simulink model "Model_6DOF"  (R2022b)
settings: Solver=VariableStepAuto  StartTime=0.0  StopTime=SimTime  RelTol=1e-6
InitFcn:
  | INIT_DATA
values from neighbouring files (symbols this model uses):
  g = 9.81    [aero_guid_dat.m]
  K_r = -0.02    [aero_guid_dat.m]
undefined symbols (not defined in the file or in its folder): a_L_c_max, a_N_c_max, b, C_bar, C_D_0, C_D_0_bar, C_D_alpha, C_D_d_e, C_L_0, C_L_0_bar, C_L_alpha, C_l_beta, C_l_d_a, C_L_d_e, C_l_d_r, C_l_p, C_L_q, C_l_r, C_m_0, C_m_alpha, C_m_d_e, C_m_q, C_n_beta, C_n_d_a, C_n_d_r, C_n_p, C_n_r, C_y_beta, C_y_d_a, C_y_d_r, C_y_p, C_y_r, d_T, da_max, da_rate_max, de_max, de_rate_max, dr_max, dr_rate_max, E, EA0, eR_0_IhI_Ih, eS_0_BE_Lh, eV_0_BE_Lh, G_cp, G_I, G_M, G_M_I, G_R, G_s, GC, I, INS_bias_f, INS_bias_omega, INS_imbalance_error, INS_scale_factor_error_f, INS_scale_factor_error_omega, k, K_beta, K_p ... (+34)
libraries: dspsrcs4 x11, matrix_library x6, simulink x5, sharedutil x3, aerolibasang x3, sharedtransform x2, simulink_extras x1, slpidlib x1
(part 2 of 2)

== system Model_6DOF/Airframe/Forces and Moments (in Body)/Gravitational Acceleration ==
  T_BL : Inport
  Constant3 : Constant  Value=g
  Gain1 : Gain  Gain=[ 0 0 1]
  Product1 : Product  Multiplication=Matrix(*)
  Reshape : Reshape  OutputDimensionality=Column vector (2-D)
  g : Outport
  wires:
  Constant3/1 -> Gain1/1
  Gain1/1 -> Reshape/1
  Product1/1 -> g/1  "Gravitational Acceleration components in body"
  Reshape/1 -> Product1/2
  T_BL/1 -> Product1/1

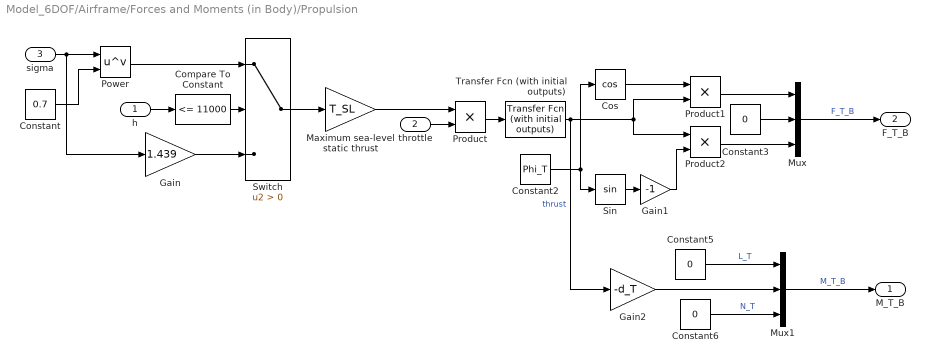
== system Model_6DOF/Airframe/Forces and Moments (in Body)/Propulsion ==
  h : Inport
  throttle : Inport  Port=2
  sigma : Inport  Port=3
  Compare To Constant : simulink/Logic and Bit Operations/Compare To Constant  relop=<=  const=11000  OutDataTypeStr=boolean
  Constant : Constant  Value=0.7
  Constant2 : Constant  Value=Phi_T
  Constant3 : Constant  Value=0
  Constant5 : Constant  Value=0
  Constant6 : Constant  Value=0
  Cos : Trigonometry  Operator=cos
  Gain : Gain  Gain=1.439
  Gain1 : Gain  Gain=-1
  Gain2 : Gain  Gain=-d_T
  Maximum sea-level static thrust : Gain  Gain=T_SL
  Mux : Mux  Inputs=3
  Mux1 : Mux  Inputs=3
  Power : Math  Operator=pow
  Product : Product
  Product1 : Product
  Product2 : Product
  Sin : Trigonometry
  Switch : Switch  Criteria=u2 > Threshold  SaturateOnIntegerOverflow=off  InputSameDT=off
  Transfer Fcn (with initial outputs) : simulink_extras/Additional Linear/Transfer Fcn (with initial outputs)  N=[1]  D=[tau_engine 1]  Y0=TI  U0=0
  M_T_B : Outport
  F_T_B : Outport  Port=2
  wires:
  throttle/1 -> Product/2
  sigma/1 -> Gain/1, Power/1
  Constant/1 -> Power/2
  Maximum sea-level static thrust/1 -> Product/1
  Product/1 -> Transfer Fcn (with initial outputs)/1
  Transfer Fcn (with initial outputs)/1 -> Product1/2, Product2/1, Gain2/1  "thrust"
  Compare To Constant/1 -> Switch/2
  Power/1 -> Switch/1
  h/1 -> Compare To Constant/1
  Switch/1 -> Maximum sea-level static thrust/1
  Gain/1 -> Switch/3
  Constant2/1 -> Sin/1, Cos/1
  Mux/1 -> F_T_B/1  "F_T_B"
  Constant3/1 -> Mux/2
  Product1/1 -> Mux/1
  Product2/1 -> Mux/3
  Cos/1 -> Product1/1
  Sin/1 -> Gain1/1
  Gain1/1 -> Product2/2
  Constant5/1 -> Mux1/1  "L_T"
  Constant6/1 -> Mux1/3  "N_T"
  Mux1/1 -> M_T_B/1  "M_T_B"
  Gain2/1 -> Mux1/2

== system Model_6DOF/Autopilot (Control system)/Acceleration Autopilot/Acceleration Autopilot ==
  a_N_c : Inport
  In Bus Element : Inport  Port=2  PortName=INS_Data  Element=f_sp_B
  In Bus Element1 : Inport  Port=2  PortName=INS_Data  Element=pqr
  Add : Sum  Inputs=+-
  Add1 : Sum  Inputs=--
  Add2 : Sum  Inputs=+-
  Gain : Gain  Gain=-g
  Gain1 : Gain  Gain=G_R
  Gain2 : Gain  Gain=G_I
  Gain3 : Gain  Gain=K_q
  Gain4 : Gain  Gain=-1
  Integrator : Integrator
  Saturation : Saturate  UpperLimit=de_max  LowerLimit=-de_max
  Saturation1 : Saturate  UpperLimit=a_N_c_max  LowerLimit=-a_N_c_max
  Saturation2 : Saturate  UpperLimit=q_c_max  LowerLimit=-q_c_max
  Selector : Selector  InputPortWidth=3  IndexOptions=Index vector (dialog)  Indices=3  OutputSizes=1
  Selector1 : Selector  InputPortWidth=3  IndexOptions=Index vector (dialog)  Indices=2  OutputSizes=1
  d_e_c : Outport
  wires:
  Gain/1 -> Add/1
  Selector/1 -> Add/2
  Add/1 -> Gain2/1, Gain1/1
  Gain2/1 -> Integrator/1
  Gain1/1 -> Add1/1
  Integrator/1 -> Add1/2
  Add2/1 -> Saturation/1
  Saturation/1 -> Gain4/1
  Saturation1/1 -> Gain/1
  Add1/1 -> Saturation2/1  "q_c"
  Saturation2/1 -> Add2/1
  a_N_c/1 -> Saturation1/1
  In Bus Element/1 -> Selector/1
  In Bus Element1/1 -> Selector1/1
  Selector1/1 -> Gain3/1  "q"
  Gain3/1 -> Add2/2
  Gain4/1 -> d_e_c/1

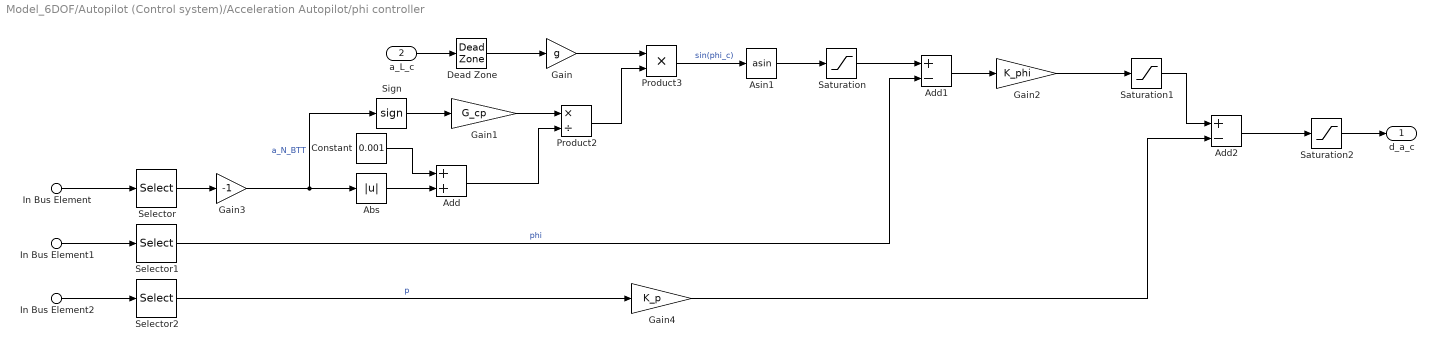
== system Model_6DOF/Autopilot (Control system)/Acceleration Autopilot/phi controller ==
  In Bus Element : Inport  PortName=INS_Data  Element=f_sp_B
  In Bus Element1 : Inport  PortName=INS_Data  Element=phi_theta_psi
  In Bus Element2 : Inport  PortName=INS_Data  Element=pqr
  a_L_c : Inport  Port=2
  Abs : Abs  SaturateOnIntegerOverflow=off
  Add : Sum
  Add1 : Sum  Inputs=+-
  Add2 : Sum  Inputs=+-
  Asin1 : Trigonometry  Operator=asin
  Constant : Constant  Value=0.001
  Dead Zone : DeadZone  LowerValue=-0.01*g  UpperValue=0.01*g
  Gain : Gain  Gain=g
  Gain1 : Gain  Gain=G_cp
  Gain2 : Gain  Gain=K_phi
  Gain3 : Gain  Gain=-1
  Gain4 : Gain  Gain=K_p
  Product2 : Product  Inputs=*/
  Product3 : Product
  Saturation : Saturate  UpperLimit=phi_c_max  LowerLimit=-phi_c_max
  Saturation1 : Saturate  UpperLimit=p_c_max  LowerLimit=-p_c_max
  Saturation2 : Saturate  UpperLimit=da_max  LowerLimit=-da_max
  Selector : Selector  InputPortWidth=3  IndexOptions=Index vector (dialog)  Indices=3  OutputSizes=1
  Selector1 : Selector  InputPortWidth=3  IndexOptions=Index vector (dialog)  Indices=1  OutputSizes=1
  Selector2 : Selector  InputPortWidth=3  IndexOptions=Index vector (dialog)  Indices=1  OutputSizes=1
  Sign : Signum
  d_a_c : Outport
  wires:
  Product3/1 -> Asin1/1  "sin(phi_c)"
  Asin1/1 -> Saturation/1
  Gain3/1 -> Sign/1, Abs/1  "a_N_BTT"
  Gain/1 -> Product3/1
  Sign/1 -> Gain1/1
  Gain1/1 -> Product2/1
  Add/1 -> Product2/2
  Dead Zone/1 -> Gain/1
  Abs/1 -> Add/2
  Product2/1 -> Product3/2
  a_L_c/1 -> Dead Zone/1
  Selector/1 -> Gain3/1
  Constant/1 -> Add/1
  In Bus Element/1 -> Selector/1
  Saturation/1 -> Add1/1
  In Bus Element1/1 -> Selector1/1
  Selector1/1 -> Add1/2  "phi"
  In Bus Element2/1 -> Selector2/1
  Add1/1 -> Gain2/1
  Gain2/1 -> Saturation1/1
  Selector2/1 -> Gain4/1  "p"
  Gain4/1 -> Add2/2
  Add2/1 -> Saturation2/1
  Saturation1/1 -> Add2/1
  Saturation2/1 -> d_a_c/1

== system Model_6DOF/Autopilot (Control system)/Mach Hold Autopilot/throttle required ==
  h : Inport
  alpha : Inport  Port=2
  M_c : Inport  Port=3
  Atmosphere : MATLAB Function  TreatAsAtomicUnit=on
  Constant : Constant  Value=C_D_0_bar
  Constant2 : Constant  Value=C_L_0_bar
  Cos : Trigonometry  Operator=cos
  "Dynamic Pressure " : aerolibasang/Dynamic Pressure
  Gain : Gain  Gain=C_L_alpha
  Gain1 : Gain  Gain=[1;0;0]
  Gain2 : Gain  Gain=k
  Gain3 : Gain  Gain=S
  Product : Product
  Product1 : Product
  Product2 : Product
  Product4 : Product  Inputs=*/
  Scope1 : Scope
  Subtract : Sum
  Subtract1 : Sum
  thrust2trrottle : Subsystem
  throttle_req : Outport
  wires:
  h/1 -> Atmosphere/1(h), thrust2trrottle/1(h)
  M_c/1 -> Product/1
  Atmosphere/2(a) -> Product/2
  Subtract1/1 -> Product1/1, Product1/2  "C_L"
  Constant2/1 -> Subtract1/2
  Constant/1 -> Subtract/1
  Gain2/1 -> Subtract/2
  Subtract/1 -> Product2/2  "C_D"
  Gain/1 -> Subtract1/1
  Product1/1 -> Gain2/1
  alpha/1 -> Cos/1, Gain/1
  Atmosphere/1(rho) -> "Dynamic Pressure "/2
  Product/1 -> Gain1/1  "V"
  "Dynamic Pressure "/1 -> Product2/1  "q"
  Gain3/1 -> Product4/1  "D"
  Cos/1 -> Product4/2
  Product4/1 -> Scope1/1, thrust2trrottle/2(thrust_req)  "thrust_req"
  thrust2trrottle/1(trottle_req) -> throttle_req/1
  Gain1/1 -> "Dynamic Pressure "/1
  Product2/1 -> Gain3/1  "D"

== system Model_6DOF/Guidance system/Optimal Guidance/t_go Calculation ==
  s_TB_L : Inport
  v_TB_L : Inport  Port=2
  Acos : Trigonometry  Operator=acos
  Constant : Constant  Value=pi/2
  Cos : Trigonometry  Operator=cos
  Divide : Product  Inputs=*/
  Divide1 : Product  Inputs=*/
  Divide2 : Product  Inputs=*/
  Dot Product : DotProduct  OutDataTypeStr=Inherit: Inherit via internal rule
  Gain : Gain  Gain=-1
  Gain3 : Gain  Gain=2
  Gain4 : Gain  Gain=2
  Product : Product
  Product1 : Product
  Sqrt : Sqrt
  Sqrt1 : Sqrt
  Square : Math  Operator=square
  Square1 : Math  Operator=square
  Subtract : Sum  Inputs=-+
  Sum of Elements : Sum  Inputs=+
  Sum of Elements1 : Sum  Inputs=+
  t_go : Outport
  wires:
  Subtract/1 -> Cos/1  "epsilon"
  Dot Product/1 -> Divide/1
  Constant/1 -> Subtract/2
  Product1/1 -> Divide2/1
  Gain/1 -> Square1/1, Dot Product/2  "v_BT_L"
  Divide/1 -> Acos/1  "cos(delta)"
  Sqrt/1 -> Product/1, Divide1/1
  Sqrt1/1 -> Product/2, Divide2/2
  Acos/1 -> Subtract/1, Gain3/1  "delta"
  Gain4/1 -> Divide1/2
  Divide1/1 -> Product1/2  "R"
  Square/1 -> Sum of Elements/1
  Square1/1 -> Sum of Elements1/1
  Sum of Elements1/1 -> Sqrt1/1
  Product/1 -> Divide/2
  s_TB_L/1 -> Square/1, Dot Product/1
  Sum of Elements/1 -> Sqrt/1
  Cos/1 -> Gain4/1
  Gain3/1 -> Product1/1  "phi"
  v_TB_L/1 -> Gain/1
  Divide2/1 -> t_go/1  "t_go"

== system Model_6DOF/INS/Accel_Triad/misalignment ==
  Constant : Constant  Value=M_a_B
  M_a_B : Outport
  wires:
  Constant/1 -> M_a_B/1

== system Model_6DOF/INS/Accel_Triad/random bias and noise ==
  Gain : Gain  Gain=INS_bias_f
  Mux : Mux  Inputs=3
  Random Source : dspsrcs4/Random Source  SrcType=Uniform  NormMethod=Ziggurat  CltLength=12  MinVal=0  MaxVal=1  MeanVal=0  VarVal=1  RepMode=Not repeatable  rawSeed=1  IsInherit=off  SampMode=Discrete  SampTime=0.1  SampFrame=1  DataType=Single  OutComplex=Real  OutputFrames=off
  Random Source1 : dspsrcs4/Random Source  SrcType=Uniform  NormMethod=Ziggurat  CltLength=12  MinVal=0  MaxVal=1  MeanVal=0  VarVal=1  RepMode=Not repeatable  rawSeed=1  IsInherit=off  SampMode=Discrete  SampTime=0.1  SampFrame=1  DataType=Single  OutComplex=Real  OutputFrames=off
  Random Source2 : dspsrcs4/Random Source  SrcType=Uniform  NormMethod=Ziggurat  CltLength=12  MinVal=0  MaxVal=1  MeanVal=0  VarVal=1  RepMode=Not repeatable  rawSeed=1  IsInherit=off  SampMode=Discrete  SampTime=0.1  SampFrame=1  DataType=Single  OutComplex=Real  OutputFrames=off
  Reshape : Reshape  OutputDimensionality=Column vector (2-D)
  e_b_a_B : Outport
  wires:
  Random Source2/1 -> Mux/3
  Random Source1/1 -> Mux/2
  Random Source/1 -> Mux/1
  Gain/1 -> Reshape/1
  Reshape/1 -> e_b_a_B/1
  Mux/1 -> Gain/1

== system Model_6DOF/INS/Accel_Triad/scale factor error ==
  Constant : Constant  Value=INS_scale_factor_error_f
  Create Diagonal Matrix : matrix_library/Create Diagonal Matrix
  S_a_B : Outport
  wires:
  Create Diagonal Matrix/1 -> S_a_B/1
  Constant/1 -> Create Diagonal Matrix/1

== system Model_6DOF/INS/Gyro_Triad/imbalance matrix ==
  Constant : Constant  Value=INS_imbalance_error
  Create Diagonal Matrix : matrix_library/Create Diagonal Matrix
  U_g_B : Outport
  wires:
  Create Diagonal Matrix/1 -> U_g_B/1
  Constant/1 -> Create Diagonal Matrix/1

== system Model_6DOF/INS/Gyro_Triad/misalignment ==
  Constant : Constant  Value=M_g_B
  M_g_B : Outport
  wires:
  Constant/1 -> M_g_B/1

== system Model_6DOF/INS/Gyro_Triad/random bias and noise ==
  Gain : Gain  Gain=INS_bias_omega
  Mux : Mux  Inputs=3
  Random Source : dspsrcs4/Random Source  SrcType=Uniform  NormMethod=Ziggurat  CltLength=12  MinVal=0  MaxVal=1  MeanVal=0  VarVal=1  RepMode=Not repeatable  rawSeed=1  IsInherit=off  SampMode=Discrete  SampTime=0.1  SampFrame=1  DataType=Single  OutComplex=Real  OutputFrames=off
  Random Source1 : dspsrcs4/Random Source  SrcType=Uniform  NormMethod=Ziggurat  CltLength=12  MinVal=0  MaxVal=1  MeanVal=0  VarVal=1  RepMode=Not repeatable  rawSeed=1  IsInherit=off  SampMode=Discrete  SampTime=0.1  SampFrame=1  DataType=Single  OutComplex=Real  OutputFrames=off
  Random Source2 : dspsrcs4/Random Source  SrcType=Uniform  NormMethod=Ziggurat  CltLength=12  MinVal=0  MaxVal=1  MeanVal=0  VarVal=1  RepMode=Not repeatable  rawSeed=1  IsInherit=off  SampMode=Discrete  SampTime=0.1  SampFrame=1  DataType=Single  OutComplex=Real  OutputFrames=off
  Reshape : Reshape  OutputDimensionality=Column vector (2-D)
  e_b_g_B : Outport
  wires:
  Random Source2/1 -> Mux/3
  Random Source1/1 -> Mux/2
  Random Source/1 -> Mux/1
  Mux/1 -> Gain/1
  Reshape/1 -> e_b_g_B/1
  Gain/1 -> Reshape/1

== system Model_6DOF/INS/Gyro_Triad/scale factor error ==
  Constant : Constant  Value=INS_scale_factor_error_omega
  Create Diagonal Matrix : matrix_library/Create Diagonal Matrix
  S_g_B : Outport
  wires:
  Create Diagonal Matrix/1 -> S_g_B/1
  Constant/1 -> Create Diagonal Matrix/1

== system Model_6DOF/Seeker/Dynamic Seeker/Radom ==
  theta_SB : Inport
  Gain : Gain  Gain=0.01
  Out1 : Outport
  wires:
  theta_SB/1 -> Gain/1
  Gain/1 -> Out1/1

== system Model_6DOF/Seeker/Dynamic Seeker/Radom  ==
  psi_SB : Inport
  Gain : Gain  Gain=0.01
  Out1 : Outport
  wires:
  psi_SB/1 -> Gain/1
  Gain/1 -> Out1/1

== system Model_6DOF/Seeker/Dynamic Seeker/Scintillation ==
  G_Scnt : Gain
  Mux : Mux  Inputs=3
  Random Source : dspsrcs4/Random Source  SrcType=Uniform  NormMethod=Ziggurat  CltLength=12  MinVal=-1  MaxVal=1  MeanVal=0  VarVal=1  RepMode=Not repeatable  rawSeed=1  IsInherit=off  SampMode=Continuous  SampTime=0.01  SampFrame=1  DataType=Double  OutComplex=Real  OutputFrames=off
  Random Source1 : dspsrcs4/Random Source  SrcType=Uniform  NormMethod=Ziggurat  CltLength=12  MinVal=-1  MaxVal=1  MeanVal=0  VarVal=1  RepMode=Not repeatable  rawSeed=1  IsInherit=off  SampMode=Continuous  SampTime=0.01  SampFrame=1  DataType=Double  OutComplex=Real  OutputFrames=off
  Random Source2 : dspsrcs4/Random Source  SrcType=Uniform  NormMethod=Ziggurat  CltLength=12  MinVal=-1  MaxVal=1  MeanVal=0  VarVal=1  RepMode=Not repeatable  rawSeed=1  IsInherit=off  SampMode=Continuous  SampTime=0.01  SampFrame=1  DataType=Double  OutComplex=Real  OutputFrames=off
  s_TO_L : Outport
  wires:
  Random Source1/1 -> Mux/2
  Random Source/1 -> Mux/1
  Random Source2/1 -> Mux/3
  G_Scnt/1 -> s_TO_L/1
  Mux/1 -> G_Scnt/1

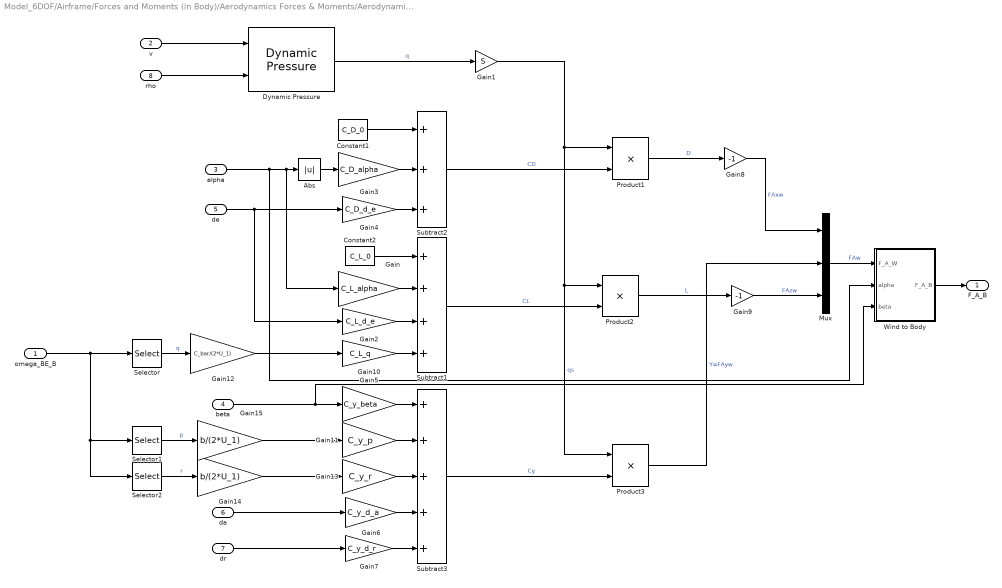
== system Model_6DOF/Airframe/Forces and Moments (in Body)/Aerodynamics Forces & Moments/Aerodynamics Forces (body) ==
  omega_BE_B : Inport
  v : Inport  Port=2
  alpha : Inport  Port=3
  beta : Inport  Port=4
  de : Inport  Port=5
  da : Inport  Port=6
  dr : Inport  Port=7
  rho : Inport  Port=8
  Abs : Abs  SaturateOnIntegerOverflow=off
  Constant1 : Constant  Value=C_D_0
  Constant2 : Constant  Value=C_L_0
  "Dynamic Pressure " : aerolibasang/Dynamic Pressure
  Gain : Gain  Gain=C_L_alpha
  Gain1 : Gain  Gain=S
  Gain10 : Gain  Gain=C_L_q
  Gain11 : Gain  Gain=C_y_p
  Gain12 : Gain  Gain=C_bar/(2*U_1)
  Gain13 : Gain  Gain=C_y_r
  Gain14 : Gain  Gain=b/(2*U_1)
  Gain15 : Gain  Gain=b/(2*U_1)
  Gain2 : Gain  Gain=C_L_d_e
  Gain3 : Gain  Gain=C_D_alpha
  Gain4 : Gain  Gain=C_D_d_e
  Gain5 : Gain  Gain=C_y_beta
  Gain6 : Gain  Gain=C_y_d_a
  Gain7 : Gain  Gain=C_y_d_r
  Gain8 : Gain  Gain=-1
  Gain9 : Gain  Gain=-1
  Mux : Mux  Inputs=3
  Product1 : Product
  Product2 : Product
  Product3 : Product
  Selector : Selector  InputPortWidth=3  IndexOptions=Index vector (dialog)  Indices=2  OutputSizes=1
  Selector1 : Selector  InputPortWidth=3  IndexOptions=Index vector (dialog)  Indices=1  OutputSizes=1
  Selector2 : Selector  InputPortWidth=3  IndexOptions=Index vector (dialog)  Indices=3  OutputSizes=1
  Subtract1 : Sum  Inputs=++++
  Subtract2 : Sum  Inputs=+++
  Subtract3 : Sum  Inputs=+++++
  Wind to Body : MATLAB Function  TreatAsAtomicUnit=on
  F_A_B : Outport
  wires:
  v/1 -> "Dynamic Pressure "/1
  "Dynamic Pressure "/1 -> Gain1/1  "q"
  Constant2/1 -> Subtract1/1
  rho/1 -> "Dynamic Pressure "/2
  Subtract1/1 -> Product2/2  "CL"
  Gain/1 -> Subtract1/2
  Gain2/1 -> Subtract1/3
  de/1 -> Gain2/1, Gain4/1
  Gain3/1 -> Subtract2/2
  Gain4/1 -> Subtract2/3
  Subtract2/1 -> Product1/2  "CD"
  Constant1/1 -> Subtract2/1
  alpha/1 -> Wind to Body/2(alpha), Abs/1, Gain/1
  Gain1/1 -> Product1/1, Product3/1, Product2/1  "qs"
  Gain5/1 -> Subtract3/1
  Gain6/1 -> Subtract3/4
  Subtract3/1 -> Product3/2  "Cy"
  Gain7/1 -> Subtract3/5
  beta/1 -> Wind to Body/3(beta), Gain5/1
  da/1 -> Gain6/1
  dr/1 -> Gain7/1
  Product1/1 -> Gain8/1  "D"
  Product2/1 -> Gain9/1  "L"
  Product3/1 -> Mux/2  "Y=FAyw"
  Mux/1 -> Wind to Body/1(F_A_W)  "FAw"
  Wind to Body/1(F_A_B) -> F_A_B/1
  Gain8/1 -> Mux/1  "FAxw"
  Gain9/1 -> Mux/3  "FAzw"
  Abs/1 -> Gain3/1
  Gain10/1 -> Subtract1/4
  omega_BE_B/1 -> Selector/1, Selector2/1, Selector1/1
  Selector/1 -> Gain12/1  "q"
  Selector1/1 -> Gain15/1  "p"
  Gain12/1 -> Gain10/1
  Gain11/1 -> Subtract3/2
  Gain13/1 -> Subtract3/3
  Selector2/1 -> Gain14/1  "r"
  Gain14/1 -> Gain13/1
  Gain15/1 -> Gain11/1

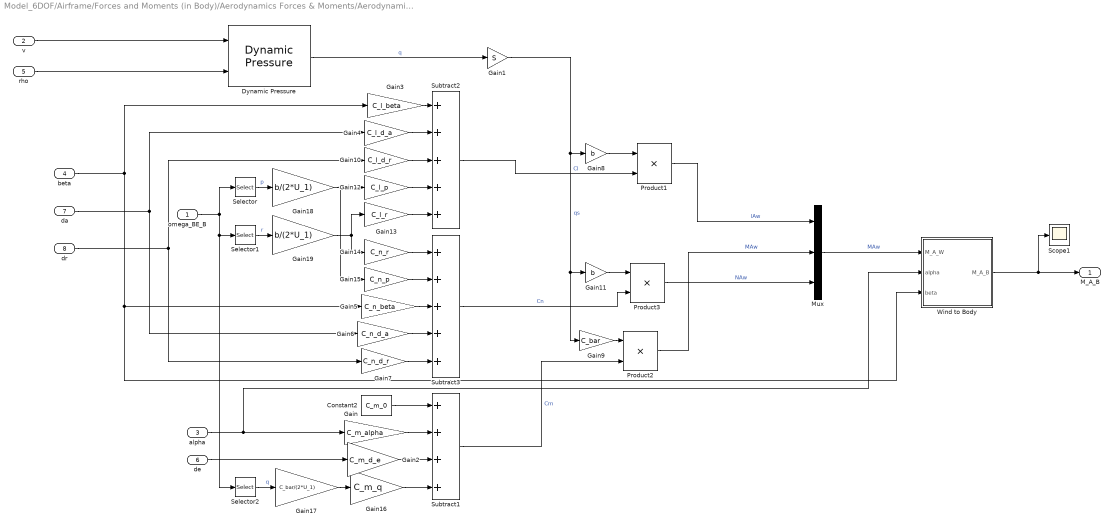
== system Model_6DOF/Airframe/Forces and Moments (in Body)/Aerodynamics Forces & Moments/Aerodynamics Moments (body) ==
  omega_BE_B : Inport
  v : Inport  Port=2
  alpha : Inport  Port=3
  beta : Inport  Port=4
  rho : Inport  Port=5
  de : Inport  Port=6
  da : Inport  Port=7
  dr : Inport  Port=8
  Constant2 : Constant  Value=C_m_0
  "Dynamic Pressure " : aerolibasang/Dynamic Pressure
  Gain : Gain  Gain=C_m_alpha
  Gain1 : Gain  Gain=S
  Gain10 : Gain  Gain=C_l_d_r
  Gain11 : Gain  Gain=b
  Gain12 : Gain  Gain=C_l_p
  Gain13 : Gain  Gain=C_l_r
  Gain14 : Gain  Gain=C_n_r
  Gain15 : Gain  Gain=C_n_p
  Gain16 : Gain  Gain=C_m_q
  Gain17 : Gain  Gain=C_bar/(2*U_1)
  Gain18 : Gain  Gain=b/(2*U_1)
  Gain19 : Gain  Gain=b/(2*U_1)
  Gain2 : Gain  Gain=C_m_d_e
  Gain3 : Gain  Gain=C_l_beta
  Gain4 : Gain  Gain=C_l_d_a
  Gain5 : Gain  Gain=C_n_beta
  Gain6 : Gain  Gain=C_n_d_a
  Gain7 : Gain  Gain=C_n_d_r
  Gain8 : Gain  Gain=b
  Gain9 : Gain  Gain=C_bar
  Mux : Mux  Inputs=3
  Product1 : Product
  Product2 : Product
  Product3 : Product
  Scope1 : Scope
  Selector : Selector  InputPortWidth=3  IndexOptions=Index vector (dialog)  Indices=1  OutputSizes=1
  Selector1 : Selector  InputPortWidth=3  IndexOptions=Index vector (dialog)  Indices=3  OutputSizes=1
  Selector2 : Selector  InputPortWidth=3  IndexOptions=Index vector (dialog)  Indices=2  OutputSizes=1
  Subtract1 : Sum  Inputs=++++
  Subtract2 : Sum  Inputs=+++++
  Subtract3 : Sum  Inputs=+++++
  Wind to Body : MATLAB Function  TreatAsAtomicUnit=on
  M_A_B : Outport
  wires:
  Product3/1 -> Mux/3  "NAw"
  Product2/1 -> Mux/2  "MAw"
  "Dynamic Pressure "/1 -> Gain1/1  "q"
  dr/1 -> Gain7/1, Gain10/1
  da/1 -> Gain6/1, Gain4/1
  beta/1 -> Gain5/1, Wind to Body/3(beta), Gain3/1
  Gain7/1 -> Subtract3/5
  Subtract2/1 -> Product1/2  "Cl"
  Gain2/1 -> Subtract1/3
  Subtract3/1 -> Product3/2  "Cn"
  Gain3/1 -> Subtract2/1
  Wind to Body/1(M_A_B) -> M_A_B/1, Scope1/1
  Gain6/1 -> Subtract3/4
  Gain/1 -> Subtract1/2
  Gain5/1 -> Subtract3/3
  Mux/1 -> Wind to Body/1(M_A_W)  "MAw"
  Subtract1/1 -> Product2/2  "Cm"
  de/1 -> Gain2/1
  Product1/1 -> Mux/1  "lAw"
  Constant2/1 -> Subtract1/1
  alpha/1 -> Wind to Body/2(alpha), Gain/1
  Gain4/1 -> Subtract2/2
  Gain10/1 -> Subtract2/3
  Gain1/1 -> Gain8/1, Gain9/1, Gain11/1  "qs"
  Gain8/1 -> Product1/1
  Gain11/1 -> Product3/1
  Gain9/1 -> Product2/1
  v/1 -> "Dynamic Pressure "/1
  rho/1 -> "Dynamic Pressure "/2
  Gain12/1 -> Subtract2/4
  omega_BE_B/1 -> Selector/1, Selector2/1, Selector1/1
  Gain13/1 -> Subtract2/5
  Selector/1 -> Gain18/1  "p"
  Gain19/1 -> Gain13/1, Gain14/1
  Gain14/1 -> Subtract3/1
  Gain15/1 -> Subtract3/2
  Selector2/1 -> Gain17/1  "q"
  Gain16/1 -> Subtract1/4
  Selector1/1 -> Gain19/1  "r"
  Gain18/1 -> Gain15/1, Gain12/1
  Gain17/1 -> Gain16/1

== system Model_6DOF/Autopilot (Control system)/Mach Hold Autopilot/throttle required/thrust2trrottle ==
  h : Inport
  thrust_req : Inport  Port=2
  Product : Product  Inputs=*/
  Saturation : Saturate  UpperLimit=1  LowerLimit=0
  max_thrust_h : Subsystem
  trottle_req : Outport
  wires:
  h/1 -> max_thrust_h/1(h)
  max_thrust_h/1(max_T_h) -> Product/2
  thrust_req/1 -> Product/1
  Product/1 -> Saturation/1
  Saturation/1 -> trottle_req/1

== system Model_6DOF/Autopilot (Control system)/Mach Hold Autopilot/throttle required/thrust2trrottle/max_thrust_h ==
  h : Inport
  Add : Sum  Inputs=+-
  Atmosphere : MATLAB Function  TreatAsAtomicUnit=on
  Constant1 : Constant  Value=11000
  Constant2 : Constant  Value=0.7
  Gain : Gain  Gain=1.439
  Gain1 : Gain  Gain=T_SL
  Power : Math  Operator=pow
  Switch : Switch  Criteria=u2 > Threshold  SaturateOnIntegerOverflow=off  InputSameDT=off
  max_T_h : Outport
  wires:
  Atmosphere/1(sigma) -> Gain/1, Power/1  "sigma"
  Gain/1 -> Switch/1
  Add/1 -> Switch/2
  Constant1/1 -> Add/2
  h/1 -> Atmosphere/1(h), Add/1
  Power/1 -> Switch/3
  Constant2/1 -> Power/2
  Switch/1 -> Gain1/1  "T/T_sl"
  Gain1/1 -> max_T_h/1

== matlab function Model_6DOF/Guidance system/Compensated PN/MATLAB Function ==
  data: T_OB output; psi_OB input; theta_OB input
function T_OB = fcn(psi_OB, theta_OB)
    T_OB = [cos(theta_OB)*cos(psi_OB) cos(theta_OB)*sin(psi_OB) -sin(theta_OB);
            -sin(psi_OB) cos(psi_OB) 0;
            sin(theta_OB)*cos(psi_OB) sin(theta_OB)*sin(psi_OB) cos(theta_OB)];

== matlab function Model_6DOF/Airframe/Atmosphere ==
  data: a output; h input; rho output; sigma output
function [a,rho,sigma] = fcn(h)
T0 = 288.15;                                     % see level temperature [k]
rho0 = 1.225;                                    % see level density [kg/m^3]
P0 = 101325;                                     % see level pressure [Pa]
rho11 = 0.3639;                                  % density at 11 km from see level [kg/m^3]
P11 = 22631.9;                                   % pressure at 11 km from see level [Pa]

if h<11000
    % Troposphere
    T = T0-0.0065*h;                                 % Temperature [k]
    theta = T/T0;                                    % Relative Temperature [-]
    rho = rho0*((T)/(T0))^4.256;                     % Density [kg/m^3]
    sigma = rho/rho0;                                % Relative Density [-]
    a = sqrt(1.4*286*T);                             % Speed of sound [m/s] sqrt(gamma*R*T)
    delta = ((T)/(T0))^5.256;                        % Relative Pressure [-]
else 
    % Stratosphere
    T = 216.65; 
    theta = T/T0;
    rho = rho11 * exp(-0.000157689*(h-11000));
    sigma = rho/rho0;
    a = sqrt(1.4*287.0531*T);
    delta = P11 * exp(-0.000157689*(h-11000))/P0;   
end

== matlab function Model_6DOF/Target ==
  data: t input; v_TE_L output size=3
function v_TE_L = fcn(t)
    v_TE_L = [100;20*sin(0.2*t);0];

== matlab function Model_6DOF/Airframe/Forces and Moments (in Body)/Aerodynamics Forces & Moments/Aerodynamics Forces (body)/Wind to Body ==
  data: F_A_W input; F_A_B output; alpha input; beta input
function F_A_B = fcn(F_A_W,alpha,beta)
    T_BW = [cos(alpha)*cos(beta) -cos(alpha)*sin(beta) -sin(alpha);
            sin(beta) cos(beta) 0;
            sin(alpha)*cos(beta) -sin(alpha)*sin(beta) cos(alpha)];
    F_A_B = T_BW*F_A_W;

== matlab function Model_6DOF/Airframe/Forces and Moments (in Body)/Aerodynamics Forces & Moments/Aerodynamics Moments (body)/Wind to Body ==
  data: M_A_W input; M_A_B output; alpha input; beta input
function M_A_B = fcn(M_A_W,alpha,beta)
    T_BW = [cos(alpha)*cos(beta) -cos(alpha)*sin(beta) -sin(alpha);
            sin(beta) cos(beta) 0;
            sin(alpha)*cos(beta) -sin(alpha)*sin(beta) cos(alpha)];
    M_A_B = T_BW*M_A_W;

== matlab function Model_6DOF/Autopilot (Control system)/Mach Hold Autopilot/throttle required/Atmosphere ==
  data: h input; rho output; a output
function [rho,a] = fcn(h)
T0 = 288.15;                                     % see level temperature [k]
rho0 = 1.225;                                    % see level density [kg/m^3]
P0 = 101325;                                     % see level pressure [Pa]
rho11 = 0.3639;                                  % density at 11 km from see level [kg/m^3]
P11 = 22631.9;                                   % pressure at 11 km from see level [Pa]

if h<11000
    % Troposphere
    T = T0-0.0065*h;                                 % Temperature [k]
    theta = T/T0;                                    % Relative Temperature [-]
    rho = rho0*((T)/(T0))^4.256;                     % Density [kg/m^3]
    a = sqrt(1.4*286*T);                             % Speed of sound [m/s] sqrt(gamma*R*T)
    delta = ((T)/(T0))^5.256;                        % Relative Pressure [-]
else 
    % Stratosphere
    T = 216.65; 
    theta = T/T0;
    rho = rho11 * exp(-0.000157689*(h-11000));   
    a = sqrt(1.4*287.0531*T);
    delta = P11 * exp(-0.000157689*(h-11000))/P0;   
end

== matlab function Model_6DOF/Seeker/Dynamic Seeker/MATLAB Function ==
  data: theta_SB input; T_SB output; psi_SB input
function T_SB = fcn(theta_SB,psi_SB)
    T_SB = [cos(psi_SB)*cos(theta_SB) sin(psi_SB) -cos(psi_SB)*sin(theta_SB);
            -sin(psi_SB)*cos(theta_SB) cos(psi_SB) sin(psi_SB)*sin(theta_SB);
            sin(theta_SB) 0 cos(theta_SB)];

== matlab function Model_6DOF/Autopilot (Control system)/Mach Hold Autopilot/throttle required/thrust2trrottle/max_thrust_h/Atmosphere ==
  data: h input; sigma output
function sigma  = fcn(h)
T0 = 288.15;                                     % see level temperature [k]
rho0 = 1.225;                                    % see level density [kg/m^3]
P0 = 101325;                                     % see level pressure [Pa]
rho11 = 0.3639;                                  % density at 11 km from see level [kg/m^3]
P11 = 22631.9;                                   % pressure at 11 km from see level [Pa]

if h<11000
    % Troposphere
    T = T0-0.0065*h;                                 % Temperature [k]
    theta = T/T0;                                    % Relative Temperature [-]
    rho = rho0*((T)/(T0))^4.256;                     % Density [kg/m^3]
    a = sqrt(1.4*286*T);                             % Speed of sound [m/s] sqrt(gamma*R*T)
    delta = ((T)/(T0))^5.256;                        % Relative Pressure [-]
    sigma = rho/rho0;                                % Relative density [-]
else 
    % Stratosphere
    T = 216.65; 
    theta = T/T0;
    rho = rho11 * exp(-0.000157689*(h-11000));   
    a = sqrt(1.4*287.0531*T);
    delta = P11 * exp(-0.000157689*(h-11000))/P0;   
    sigma = rho/rho0;
end

== matlab function Model_6DOF/Guidance system/Compensated PN/CPN ==
  data: a_m input; a_PN_O input; a_G_B_23 output; psi_OB input; theta_OB input
function a_G_B_23 = fcn(a_m,a_PN_O,psi_OB, theta_OB)
a_G_O_23 = a_PN_O(2:3) - a_m*[-sin(psi_OB);sin(theta_OB)*cos(psi_OB)];
M_1 = [sec(psi_OB) 0;
       -tan(psi_OB)*tan(theta_OB) sec(theta_OB)];
a_G_B_23 = M_1*a_G_O_23;
